simulink model "DR_S"  (R2024b)
settings: Solver=VariableStepAuto  StartTime=0.0  StopTime=10.0  MaxStep=0.01  RelTol=1e-3
InitFcn:
  | m = 10;
  | k = 100;
  | r = 0.05;

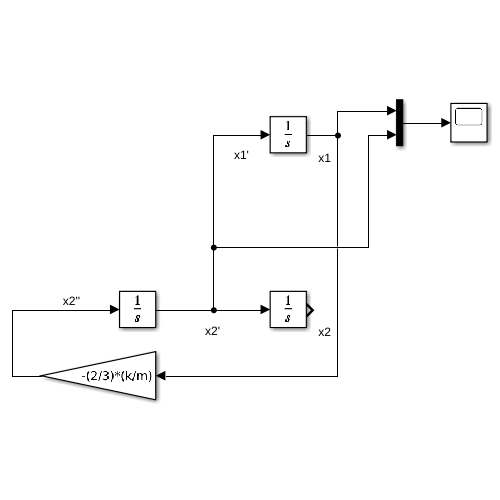
[thumbnail: Simulink's stored preview of the top-level diagram]
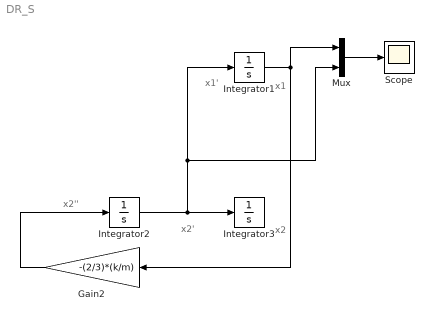
== system DR_S ==
  note: x1'
  note: x1
  note: x2''
  note: x2
  note: x2'
  Gain2 : Gain  Gain=-(2/3)*(k/m)
  Integrator1 : Integrator
  Integrator2 : Integrator  InitialCondition=2
  Integrator3 : Integrator
  Mux : Mux  Inputs=2
  Scope : Scope
  wires:
  Integrator2/1 -> Integrator3/1, Mux/2, Integrator1/1
  Integrator1/1 -> Gain2/1, Mux/1
  Mux/1 -> Scope/1
  Gain2/1 -> Integrator2/1
